simulink model "dspilbclib"  (R2020a)
settings: Solver=FixedStepDiscrete  StartTime=0.0  StopTime=inf  RelTol=1e-3  EnableMultiTasking=on
InitFcn:
  | ilbcDatatype = get_param([bdroot '/Configuration'],'ilbcDialogDatatype');
  | if strcmp(get_param([bdroot '/Configuration'],'ilbcDialogMode'), '13.33 kbit/sec mode')
  |   ilbcMode = 1;
  | else
  |   ilbcMode = 2;
  | end
model workspace: external: MAT-File dspilbcdata.mat (data not in the file)
undefined symbols (not defined in the file or in its folder): ilbc, Newton, Raphson
libraries: simulink x33, dspmtrx3 x28, dspquant2 x9, dspilbclib x8, dspstat3 x8, dspsigops x7, simulink_need_slupdate x3, dspsrcs4 x2, dspsnks4 x1, dspvision x1, dspmisc x1, dsplp x1
(part 3 of 3)

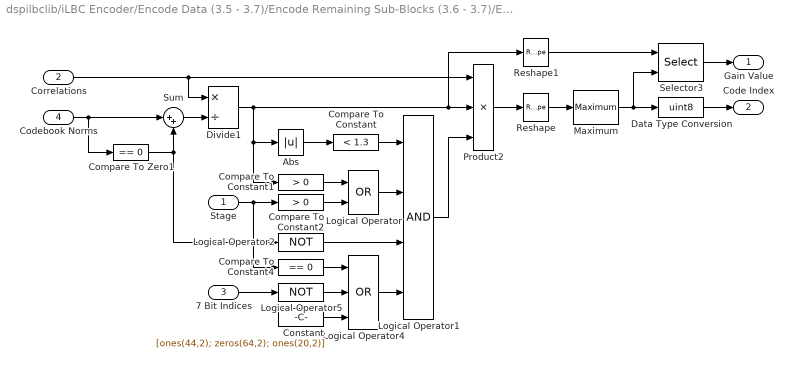
== system dspilbclib/iLBC Encoder/Encode Data (3.5 - 3.7)/Encode Remaining Sub-Blocks (3.6 - 3.7)/Encode Sub-Block (3.6.2 - 3.7)/3 Stage Sub-Block Encoder (3.6.4)/Search Codebooks (3.6.4.1 continued) ==
  Stage : Inport
  Correlations : Inport  Port=2
  7 Bit Indices : Inport  Port=3
  Codebook Norms : Inport  Port=4
  Abs : Abs
  Compare To Constant : simulink/Logic and Bit Operations/Compare To Constant  relop=<  const=1.3  OutDataTypeStr=boolean  ZeroCross=off
  Compare To Constant1 : simulink/Logic and Bit Operations/Compare To Constant  relop=>  const=0  OutDataTypeStr=boolean  ZeroCross=off
  Compare To Constant2 : simulink/Logic and Bit Operations/Compare To Constant  relop=>  const=0  OutDataTypeStr=boolean  ZeroCross=off
  Compare To Constant4 : simulink/Logic and Bit Operations/Compare To Constant  relop===  const=0  OutDataTypeStr=boolean  ZeroCross=off
  Compare To Zero1 : simulink/Logic and Bit Operations/Compare To Zero  relop===  OutDataTypeStr=boolean  ZeroCross=off
  Constant : Constant  Value=[ones(44,2); zeros(64,2); ones(20,2)]  VectorParams1D=off  OutDataTypeStr=Inherit: Inherit via back propagation
  Data Type Conversion : DataTypeConversion  OutDataTypeStr=uint8
  Divide1 : Product  Inputs=*/  OutDataTypeStr=Inherit: Same as first input
  Logical Operator : Logic  Operator=OR  AllPortsSameDT=off  OutDataTypeStr=boolean
  Logical Operator1 : Logic  Inputs=4  AllPortsSameDT=off  OutDataTypeStr=boolean
  Logical Operator2 : Logic  Operator=NOT  AllPortsSameDT=off  OutDataTypeStr=boolean
  Logical Operator4 : Logic  Operator=OR  Inputs=3  AllPortsSameDT=off  OutDataTypeStr=boolean
  Logical Operator5 : Logic  Operator=NOT  AllPortsSameDT=off  OutDataTypeStr=boolean
  Maximum : dspstat3/Maximum  operation=maximum  fcn=Index  indexBase=Zero  operateOver=Each column  Dimension=1  InputProcessing=Columns as channels (frame based)  reset=None  roiEnable=off  roiType=Rectangles  roiPortion=Entire ROI  roiOutput=Individual statistics for each ROI  roiFlag=off  roundingMode=Floor  overflowMode=off  accumDataTypeStr=Inherit: Same as product output  accumLastDataTypeStr=Inherit: Same as product output
  Product2 : Product  Inputs=3  RndMeth=Zero  OutDataTypeStr=Inherit: Same as first input
  Reshape : Reshape  OutputDimensionality=Column vector (2-D)
  Reshape1 : Reshape  OutputDimensionality=Column vector (2-D)
  Selector3 : Selector  NumberOfDimensions=2  IndexMode=Zero-based  InputPortWidth=3  IndexOptions=Index vector (port),Select all  Indices=1,1  OutputSizes=1,1
  Sum : Sum  Inputs=|++  OutDataTypeStr=Inherit: Same as first input
  Gain Value : Outport
  Code Index : Outport  Port=2
  wires:
  Divide1/1 -> Compare To Constant1/1, Abs/1, Reshape1/1, Product2/2
  Logical Operator1/1 -> Product2/3
  Logical Operator2/1 -> Logical Operator1/3
  Logical Operator/1 -> Logical Operator1/2
  Compare To Constant2/1 -> Logical Operator/2
  Compare To Constant1/1 -> Logical Operator/1
  Constant/1 -> Logical Operator4/3
  Logical Operator5/1 -> Logical Operator4/2
  Compare To Constant4/1 -> Logical Operator4/1
  Reshape1/1 -> Selector3/1
  Reshape/1 -> Maximum/1
  Stage/1 -> Compare To Constant4/1, Compare To Constant2/1
  7 Bit Indices/1 -> Logical Operator5/1
  Logical Operator4/1 -> Logical Operator1/4
  Compare To Constant/1 -> Logical Operator1/1
  Correlations/1 -> Product2/1, Divide1/1
  Maximum/1 -> Selector3/2, Data Type Conversion/1
  Compare To Zero1/1 -> Logical Operator2/1, Sum/2
  Sum/1 -> Divide1/2
  Selector3/1 -> Gain Value/1
  Product2/1 -> Reshape/1
  Data Type Conversion/1 -> Code Index/1
  Codebook Norms/1 -> Sum/1, Compare To Zero1/1
  Abs/1 -> Compare To Constant/1

== system dspilbclib/iLBC Encoder/Encode Data (3.5 - 3.7)/Encode Remaining Sub-Blocks (3.6 - 3.7)/Encode Sub-Block (3.6.2 - 3.7)/Compute Codebooks (3.6.2 - 3.6.3)/Augment Codebooks (3.6.3.3) ==
  Codebooks : Inport
  Enable : EnablePort
  Compute Augmented CB : Subsystem  TreatAsAtomicUnit=on
  Matrix Scaling1 : dspmtrx3/Array-Vector Multiply  mode=Mute  saveAsFlag=0  Dimension=1  V_Source=Dialog parameter  V_VectFromMask=[1 0.8 0.6 0.4 0.2]  roundingMode=Floor  overflowMode=off  firstCoeffSignedness=Auto  firstCoeffDataTypeStr=Inherit: Same word length as input  firstCoeffMin=[]  firstCoeffMax=[]  firstCoeffLastDataTypeStr=Inherit: Same word length as input  prodOutputSignedness=Auto  accumSignedness=Auto  outputSignedness=Auto  outputDataTypeStr=Inherit: Same as product output  outputMin=[]  outputMax=[]  outputLastDataTypeStr=Inherit: Same as product output
      settings: SourceProductBaseCode=DS
  Selector3 : Selector  NumberOfDimensions=2  InputPortWidth=3  IndexOptions=Index vector (dialog),Select all  Indices=[143:147],1  OutputSizes=1,1
  Augmented : Outport  OutputWhenDisabled=reset  InitialOutput=zeros(20,40,2)
  wires:
  Compute Augmented CB/1(Augmented) -> Augmented/1
  Codebooks/1 -> Compute Augmented CB/1(Codebook), Selector3/1
  Matrix Scaling1/1 -> Compute Augmented CB/2(Interpolation)
  Selector3/1 -> Matrix Scaling1/1

== system dspilbclib/iLBC Encoder/Encode Data (3.5 - 3.7)/Encode Remaining Sub-Blocks (3.6 - 3.7)/Encode Sub-Block (3.6.2 - 3.7)/Compute Codebooks (3.6.2 - 3.6.3)/tp00af6ee5_fd7c_4add_bbb5_3302ee0df652 ==
  in : Inport
  den : Inport  Port=2
  Scale Denominator : Product  Inputs=*/
  Scale in : Product  Inputs=*/
  Select a0 : dspmtrx3/Submatrix  RowSpan=Range of rows  RowStartMode=First  RowStartIndex=1  RowEndMode=Index  RowEndIndex=1  ColSpan=Range of columns  ColStartMode=First  ColStartIndex=1  ColEndMode=Index  ColEndIndex=1
  scaled in : Outport
  scaled den : Outport  Port=2
  wires:
  den/1 -> Select a0/1, Scale Denominator/1
  in/1 -> Scale in/1
  Select a0/1 -> Scale in/2, Scale Denominator/2
  Scale in/1 -> scaled in/1
  Scale Denominator/1 -> scaled den/1

== system dspilbclib/iLBC Encoder/Encode Data (3.5 - 3.7)/Encode Remaining Sub-Blocks (3.6 - 3.7)/Encode Sub-Block (3.6.2 - 3.7)/Compute Codebooks (3.6.2 - 3.6.3)/Augment Codebooks (3.6.3.3)/Compute Augmented CB ==
  Codebook : Inport
  Interpolation : Inport  Port=2
  Assignment1 : Assignment  NumberOfDimensions=3  OutputInitialize=Specify size for each dimension in table  IndexOptions=Index vector (port),Assign all,Assign all  Indices=1,1,1  OutputSizes=20,40,2
  Bias : Bias  Bias=15
  Compute Code : Subsystem
  Constant : Constant  Value=ilbc.augmented_idxTbl  VectorParams1D=off  OutDataTypeStr=uint8
  For Iterator : ForIterator  IterationLimit=20  IterationVariableDataType=int8
  Matrix Scaling : dspmtrx3/Array-Vector Multiply  mode=Mute  saveAsFlag=0  Dimension=1  V_Source=Dialog parameter  V_VectFromMask=[0 0.2 0.4 0.6 0.8]  roundingMode=Floor  overflowMode=off  firstCoeffSignedness=Auto  firstCoeffDataTypeStr=Inherit: Same word length as input  firstCoeffMin=[]  firstCoeffMax=[]  firstCoeffLastDataTypeStr=Inherit: Same word length as input  prodOutputSignedness=Auto  accumSignedness=Auto  outputSignedness=Auto  outputDataTypeStr=Inherit: Same as product output  outputMin=[]  outputMax=[]  outputLastDataTypeStr=Inherit: Same as product output
      settings: SourceProductBaseCode=DS
  Reshape : Reshape  OutputDimensionality=Customize  OutputDimensions=[1 40 2]
  Selector1 : Selector  NumberOfDimensions=2  InputPortWidth=3  IndexOptions=Index vector (port),Select all  Indices=[1 3],1  OutputSizes=1,1
  Selector2 : Selector  NumberOfDimensions=2  InputPortWidth=3  IndexOptions=Starting index (port),Select all  Indices=[1 3],1  OutputSizes=5,1
  Selector3 : Selector  NumberOfDimensions=2  InputPortWidth=3  IndexOptions=Select all,Index vector (port)  Indices=[1 3],1  OutputSizes=1,1
  Sum : Sum  Inputs=++|
  Augmented : Outport
  wires:
  Constant/1 -> Selector3/1
  Reshape/1 -> Assignment1/1
  Assignment1/1 -> Augmented/1
  Interpolation/1 -> Sum/1
  Matrix Scaling/1 -> Sum/2
  Selector3/1 -> Selector1/2
  Selector1/1 -> Compute Code/1(Y0), Selector2/1
  Bias/1 -> Compute Code/3(Idx1), Selector2/2
  Selector2/1 -> Matrix Scaling/1
  Codebook/1 -> Selector1/1
  For Iterator/1 -> Selector3/2, Assignment1/2, Bias/1
  Compute Code/1(Y) -> Reshape/1
  Sum/1 -> Compute Code/2(U)

== system dspilbclib/iLBC Encoder/Encode Data (3.5 - 3.7)/Encode Remaining Sub-Blocks (3.6 - 3.7)/Encode Sub-Block (3.6.2 - 3.7)/Compute Codebooks (3.6.2 - 3.6.3)/Augment Codebooks (3.6.3.3)/Compute Augmented CB/Compute Code ==
  Y0 : Inport
  U : Inport  Port=2
  Idx1 : Inport  Port=3
  Assignment : Assignment  NumberOfDimensions=2  IndexOptions=Starting index (port),Assign all  Indices=1,1  OutputSizes=40,1
  Used for reset feature only : ForIterator  ResetStates=reset  IterationLimit=1  ShowIterationPort=off  IterationVariableDataType=int8
  Y : Outport
  wires:
  Assignment/1 -> Y/1
  U/1 -> Assignment/2
  Idx1/1 -> Assignment/3
  Y0/1 -> Assignment/1
